simulink model "mech_cambelt"  (R2017b)
settings: Solver=ode5  StartTime=0.0  StopTime=5  FixedStep=0.01  RelTol=1e-3  EnableMultiTasking=on
undefined symbols (not defined in the file): m, rad, s, sigbuilder_block
libraries: mblibv1 x16
Description:
  | Cam Belt
  | 
  | This example shows a body rotating with a cam and a belt coupled to a pulley.
  | 
  | 
  | Copyright 2008-2017 The MathWorks, Inc.
settings Model: FPTRunName=Active  ExtModeAutoUpdateStatusClock=off  Creator=MathWorks  LastModifiedBy=smiller
settings DataIOCC: LimitDataPoints=on  SaveFormat=Array  SignalLoggingSaveFormat=ModelDataLogs  SignalLoggingName=sigsOut  OutputOption=SpecifiedOutputTimes  OutputTimes=[0:0.1:10]
settings OptimizationCC: ExpressionDepthLimit=2147483647  InitFltsAndDblsToZero=on  LifeSpan=inf
settings DebuggingCC: SaveWithParameterizedLinksMsg=none  UnderspecifiedInitializationDetection=Classic  MergeDetectMultiDrivingBlocksExec=none  CheckExecutionContextPreStartOutputMsg=on  CheckExecutionContextRuntimeOutputMsg=on  SignalResolutionControl=TryResolveAllWithWarning  MultiTaskDSMMsg=warning  MultiTaskCondExecSysMsg=none  SigSpecEnsureSampleTimeMsg=none  FcnCallInpInsideContextMsg=warning  StateNameClashWarn=warning  StrictBusMsg=None  SFUnexpectedBacktrackingDiag=warning  SFNoUnconditionalDefaultTransitionDiag=warning  SFExecutionAtInitializationDiag=none
settings HardwareCC: ProdBitPerPointer=32  ProdBitPerSizeT=32  ProdBitPerPtrDiffT=32  ProdLargestAtomicFloat=None  ProdIntDivRoundTo=Undefined  ProdEndianess=Unspecified  ProdWordSize=32  ProdHWDeviceType=32-bit Generic  TargetBitPerPointer=64  TargetBitPerSizeT=64  TargetBitPerPtrDiffT=64  TargetLongLongMode=on  TargetIntDivRoundTo=Zero  TargetEndianess=LittleEndian  TargetWordSize=64  TargetHWDeviceType=MATLAB Host  ProdEqTarget=off
settings ModelReferenceCC: PropagateSignalLabelsOutOfModel=off
settings RTWCC: Description=Generic Real-Time Target
settings CodeAppCC: StateflowObjectComments=on
settings GRTTargetCC: TargetLangStandard=C89/C90 (ANSI)  GeneratePreprocessorConditionals=Disable all  CombineOutputUpdateFcns=off  GRTInterface=on
settings ConfigComp: CovMetricSettings=dw  CovHtmlReporting=on  CovSaveCumulativeToWorkspaceVar=on  CovSaveSingleToWorkspaceVar=on  CovExternalEMLEnable=off
settings SimscapeCC: SimscapeNormalizeSystem=off
settings SimMechanicsCC: WarnOnRedundantConstraints=off  VisOnUpdateDiagram=on  VisDuringSimulation=on  VisConfigFile=mech_cambelt.mat
settings ConfigurationSet: Description=SimMechanics 2G

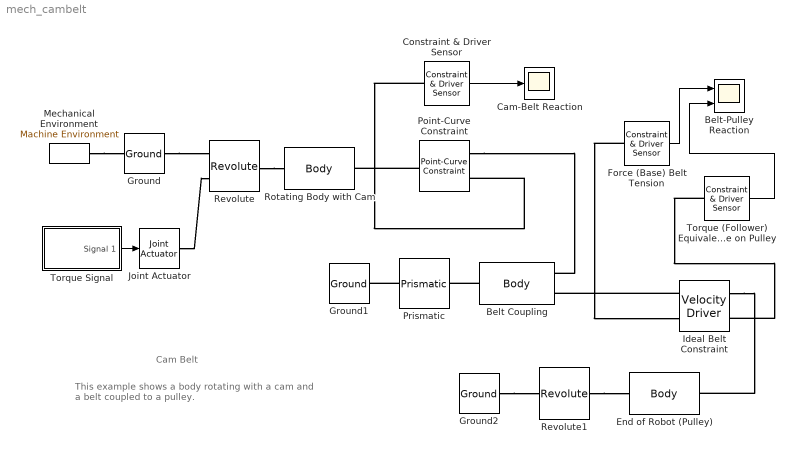
== system mech_cambelt ==
  note: Cam Belt
  note: This example shows a body rotating with a cam
      | and a belt coupled to a pulley.
  Belt Coupling : mblibv1/Bodies/Body  LConnTagsString=CS1  RConnTagsString=CS2|CS3  UpdateFromCAD=off  DialogClass=MechanicalBodyBlock  Mass=1  MassUnits=kg  InertiaUnits=kg*m^2  Inertia=(2/5)*1*[0.02 0 0;0 1 0;0 0 1]  Shape=Cylinder  ShapeDims=[1 1]  ShapeUnits=m  ShapeUse=false  Density=1  DensityUnits=kg/m^3  DensityUse=false  GraphicsMode=MACHINE_DEFAULT  BodyColorSelMode=MACHINE_DEFAULT  BodyColor=[1;0;0]  AttachedToCS=CG  CG=Left$CG$[2 0 0]$WORLD$WORLD$m$[0 0 0]$Euler X-Y-Z$deg$WORLD$false  WorkingFrames=Left$CS1$[3 0 0]$WORLD$WORLD$m$[0 0 0]$Euler X-Y-Z$deg$WORLD$true#Right$CS2$[1 0 0]$WORLD$WORLD$m$[0 0 0]$Euler X-Y-Z$deg$WORLD$true#Right$CS3$[1 0 0]$WORLD$WORLD$m$[0 0 0]$Euler X-Y-Z$deg$WORLD$true  CGPos=[2 0 0]  CGRot=[0 0 0]  CS0Pos=[]  CS0Rot=[]  CS1Pos=[3 0 0]  CS1Rot=[0 0 0]  CS2Pos=[1 0 0]  CS2Rot=[0 0 0]  CS3Pos=[1 0 0]  CS3Rot=[0 0 0]  CS4Pos=[]  CS4Rot=[]  CS5Pos=[]  CS5Rot=[]  CS6Pos=[]  CS6Rot=[]  CS7Pos=[]  CS7Rot=[]  CS8Pos=[]  CS8Rot=[]  CS9Pos=[]  CS9Rot=[]  CS10Pos=[]  CS10Rot=[]  CS11Pos=[]  CS11Rot=[]  CS12Pos=[]  CS12Rot=[]  CS13Pos=[]  CS13Rot=[]  CS14Pos=[]  CS14Rot=[]  CS15Pos=[]  CS15Rot=[]  CS16Pos=[]  CS16Rot=[]  CS17Pos=[]  CS17Rot=[]  CS18Pos=[]  CS18Rot=[]  CS19Pos=[]  CS19Rot=[]  CS20Pos=[]  CS20Rot=[]
      settings: SourceProductName=Simscape Multibody  SourceProductBaseCode=MS
  Belt-Pulley Reaction : Scope  NumInputPorts=2
  Cam-Belt Reaction : Scope
  Constraint & Driver Sensor : mblibv1/Sensors &  Actuators/Constraint & Driver  Sensor  UpdateFromCAD=off  LeftPortType=blob  RightPortType=blob  PhysicalDomain=Mechanical  DialogClass=ConstraintSensorBlock  SensedSide=Base  ReferenceFrame=Absolute (World)  ReactionForce=on  ForceUnits=N  ReactionMoment=on  MomentUnits=N-m  Muxed=on  OutputVector=[ 3 3 ]  ActiveIO=on  Width=6
      settings: SourceProductName=Simscape Multibody  SourceProductBaseCode=MS
  End of Robot (Pulley) : mblibv1/Bodies/Body  LConnTagsString=CS1  RConnTagsString=CS2  UpdateFromCAD=off  DialogClass=MechanicalBodyBlock  Mass=1  MassUnits=kg  InertiaUnits=kg*m^2  Inertia=(2/5)*1*[0.5 0 0;0 0.5 0;0 0 1]  Shape=Cylinder  ShapeDims=[1 1]  ShapeUnits=m  ShapeUse=false  Density=1  DensityUnits=kg/m^3  DensityUse=false  GraphicsMode=MACHINE_DEFAULT  BodyColorSelMode=MACHINE_DEFAULT  BodyColor=[1;0;0]  AttachedToCS=CG  CG=Left$CG$[0 0 0]$CS1$CS1$m$[0 0 0]$Euler X-Y-Z$deg$WORLD$false  WorkingFrames=Left$CS1$[0 0 0]$ADJOINING$ADJOINING$m$[0 0 0]$Euler X-Y-Z$deg$WORLD$true#Right$CS2$[0 0 0]$CS1$CS1$m$[0 0 0]$Euler X-Y-Z$deg$WORLD$true#Right$CS3$[0 1 0]$CS1$CS1$m$[0 0 0]$Euler X-Y-Z$deg$WORLD$false#Right$CS4$[-1 0 0]$CS1$CS1$m$[0 0 0]$Euler X-Y-Z$deg$WORLD$false#Right$CS5$[0 -1 0]$CS1$CS1$m$[0 0 0]$Euler X-Y-Z$deg$WORLD$false#Right$CS6$[1 0 0]$CS1$CS1$m$[0 0 0]$Euler X-Y-Z$deg$WORLD$false  CGPos=[0 0 0]  CGRot=[0 0 0]  CS0Pos=[]  CS0Rot=[]  CS1Pos=[0 0 0]  CS1Rot=[0 0 0]  CS2Pos=[0 0 0]  CS2Rot=[0 0 0]  CS3Pos=[0 1 0]  CS3Rot=[0 0 0]  CS4Pos=[-1 0 0]  CS4Rot=[0 0 0]  CS5Pos=[0 -1 0]  CS5Rot=[0 0 0]  CS6Pos=[1 0 0]  CS6Rot=[0 0 0]  CS7Pos=[]  CS7Rot=[]  CS8Pos=[]  CS8Rot=[]  CS9Pos=[]  CS9Rot=[]  CS10Pos=[]  CS10Rot=[]  CS11Pos=[]  CS11Rot=[]  CS12Pos=[]  CS12Rot=[]  CS13Pos=[]  CS13Rot=[]  CS14Pos=[]  CS14Rot=[]  CS15Pos=[]  CS15Rot=[]  CS16Pos=[]  CS16Rot=[]  CS17Pos=[]  CS17Rot=[]  CS18Pos=[]  CS18Rot=[]  CS19Pos=[]  CS19Rot=[]  CS20Pos=[]  CS20Rot=[]
      settings: SourceProductName=Simscape Multibody  SourceProductBaseCode=MS
  Force (Base) Belt Tension : mblibv1/Sensors &  Actuators/Constraint & Driver  Sensor  UpdateFromCAD=off  LeftPortType=blob  RightPortType=blob  PhysicalDomain=Mechanical  DialogClass=ConstraintSensorBlock  SensedSide=Base  ReferenceFrame=Absolute (World)  ReactionForce=on  ForceUnits=N  ReactionMoment=off  MomentUnits=N-m  Muxed=on  OutputVector=[ 3 ]  ActiveIO=on  Width=3
      settings: SourceProductName=Simscape Multibody  SourceProductBaseCode=MS
  Ground : mblibv1/Bodies/Ground  UpdateFromCAD=off  LeftPortType=env  RightPortType=workingframe  PhysicalDomain=Mechanical  DialogClass=GroundBlock  CoordPosition=[0 0 0]  CoordPositionUnits=m  StateVectorMgrId=-1  MachineId=[0 0]  ShowEnvPort=on  ParameterChecksum=[0 0 0 0]  TopologyChecksum=[0 0 0 0]
      settings: SourceProductName=Simscape Multibody  SourceProductBaseCode=MS
  Ground1 : mblibv1/Bodies/Ground  UpdateFromCAD=off  LeftPortType=env  RightPortType=workingframe  PhysicalDomain=Mechanical  DialogClass=GroundBlock  CoordPosition=[3 0 0]  CoordPositionUnits=m  StateVectorMgrId=-1  MachineId=[0 0]  ShowEnvPort=off  ParameterChecksum=[0 0 0 0]  TopologyChecksum=[0 0 0 0]
      settings: SourceProductName=Simscape Multibody  SourceProductBaseCode=MS
  Ground2 : mblibv1/Bodies/Ground  UpdateFromCAD=off  LeftPortType=env  RightPortType=workingframe  PhysicalDomain=Mechanical  DialogClass=GroundBlock  CoordPosition=[5 2 0]  CoordPositionUnits=m  StateVectorMgrId=-1  MachineId=[0 0]  ShowEnvPort=off  ParameterChecksum=[0 0 0 0]  TopologyChecksum=[0 0 0 0]
      settings: SourceProductName=Simscape Multibody  SourceProductBaseCode=MS
  Ideal Belt Constraint : mblibv1/Constraints &  Drivers/Velocity Driver  LConnTagsString=__newl0|SA1  RConnTagsString=__newr0|SA1  UpdateFromCAD=off  DialogClass=ConstantVelocityConstraint  NumSAPorts=2  Unit_V=m/s  Unit_Omega=rad/s  Coef_V_Base=[1 0 0]  Csys_V_Base=WORLD  Coef_Omega_Base=[0 0 0]  Csys_Omega_Base=WORLD  Coef_V_Follower=[0 0 0]  Csys_V_Follower=WORLD  Coef_Omega_Follower=[0 0 1]  Csys_Omega_Follower=WORLD
      settings: SourceProductName=Simscape Multibody  SourceProductBaseCode=MS
  Joint Actuator : mblibv1/Sensors &  Actuators/Joint Actuator  UpdateFromCAD=off  PhysicalDomain=Mechanical  PortType=blob  ActuationStyle=Force  AngleUnits=deg  ArcVelocityUnits=deg/s  ArcAccelerationUnits=deg/s^2  CoordPositionUnits=m  VelocityUnits=m/s  AccelerationUnits=m/s^2  ForceUnits=N  TorqueUnits=N-m  ActiveIO=on  Width=1  DialogClass=MechanicalActuatorBlock  Primitive=R1  ReferenceFrame=Absolute (INERTIAL)
      settings: SourceProductName=Simscape Multibody  SourceProductBaseCode=MS
  Mechanical Environment : mblibv1/Bodies/Machine Environment  Tag=Factory ground  PortType=env  PhysicalDomain=Mechanical  DialogTemplateClass=MECH.MachineEnvironment  SyncWhenCopied=off  Gravity=[0 -9.81 0]  GravityUnits=m/s^2  GravityAsSignal=off  Dimensionality=3D Only  AnalysisType=Forward dynamics  LinearAssemblyTolerance=1e-3  LinearAssemblyToleranceUnits=m  AngularAssemblyTolerance=1e-3  AngularAssemblyToleranceUnits=rad  ConstraintSolverType=Stabilizing  ConstraintRelTolerance=1e-4  ConstraintAbsTolerance=1e-4  UseRobustSingularityHandling=off  RedundancyAnalysisToleranceType=Automatically select tolerance  RedundancyAnalysisTolerance=1e-14  StatePerturbationType=Fixed  PerturbationSize=1e-5  VisualizeMachine=on  BodyVisualizationType=Use model default body geometries  BodyColorSelMode=Use model default  DefaultBodyColor=[1 0 0]
      settings: SourceProductName=Simscape Multibody  SourceProductBaseCode=MS
  Point-Curve Constraint : mblibv1/Constraints &  Drivers/Point-Curve Constraint  LConnTagsString=__newl0|SA1  RConnTagsString=__newr0  UpdateFromCAD=off  DialogClass=PointCurveConstraint  Units=m  Xbreaks="[1     0.77547    0.058989    -0.52528    -0.55899    -0.17022     0.65485]"  Ybreaks="[0     0.42955     0.56832     0.29503    -0.12733    -0.36512    -0.39199]"  Zbreaks="[-0.0031056     0.36957     0.56832     0.29503    -0.12733    -0.46273    -0.40062]*0"  EndConditions=periodic  CanExtrapolate=off  NumSAPorts=1
      settings: SourceProductName=Simscape Multibody  SourceProductBaseCode=MS
  Prismatic : mblibv1/Joints/Prismatic  LConnTagsString=__newl0  RConnTagsString=__newr0  UpdateFromCAD=off  NumSAPorts=0  CutJoint=off  MarkAsCut=off  Primitives=prismatic  PrimitiveProps=P1$WORLD$[-1 0 0]$prismatic  DialogClass=JointBlock  P1Axis=[-1 0 0]
      settings: SourceProductName=Simscape Multibody  SourceProductBaseCode=MS
  Revolute : mblibv1/Joints/Revolute  LConnTagsString=__newl0|SA1  RConnTagsString=__newr0  UpdateFromCAD=off  NumSAPorts=1  CutJoint=off  MarkAsCut=off  Primitives=revolute  PrimitiveProps=R1$WORLD$[0 0 1]$revolute  DialogClass=JointBlock  R1Axis=[0 0 1]
      settings: SourceProductName=Simscape Multibody  SourceProductBaseCode=MS
  Revolute1 : mblibv1/Joints/Revolute  LConnTagsString=__newl0  RConnTagsString=__newr0  UpdateFromCAD=off  NumSAPorts=0  CutJoint=off  MarkAsCut=off  Primitives=revolute  PrimitiveProps=R1$WORLD$[0 0 1]$revolute  DialogClass=JointBlock  R1Axis=[0 0 1]
      settings: SourceProductName=Simscape Multibody  SourceProductBaseCode=MS
  Rotating Body with Cam : mblibv1/Bodies/Body  LConnTagsString=CS1  RConnTagsString=CS2  UpdateFromCAD=off  DialogClass=MechanicalBodyBlock  Mass=1  MassUnits=kg  InertiaUnits=kg*m^2  Inertia=(2/5)*1*[0.5 0 0;0 0.5 0;0 0 1]  Shape=Cylinder  ShapeDims=[1 1]  ShapeUnits=m  ShapeUse=false  Density=1  DensityUnits=kg/m^3  DensityUse=false  GraphicsMode=MACHINE_DEFAULT  BodyColorSelMode=MACHINE_DEFAULT  BodyColor=[1;0;0]  AttachedToCS=CG  CG=Left$CG$[0 0 0]$WORLD$WORLD$m$[0 0 0]$Euler X-Y-Z$deg$WORLD$false  WorkingFrames=Left$CS1$[0 0 0]$WORLD$WORLD$m$[0 0 0]$Euler X-Y-Z$deg$WORLD$true#Right$CS2$[0 0 0]$CS1$CS1$m$[0 0 0]$Euler X-Y-Z$deg$WORLD$true#Right$CS3$[0 1 0]$CS1$CS1$m$[0 0 0]$Euler X-Y-Z$deg$WORLD$false#Right$CS4$[-1 0 0]$CS1$CS1$m$[0 0 0]$Euler X-Y-Z$deg$WORLD$false#Right$CS5$[0 -1 0]$CS1$CS1$m$[0 0 0]$Euler X-Y-Z$deg$WORLD$false#Right$CS6$[1 0 0]$CS1$CS1$m$[0 0 0]$Euler X-Y-Z$deg$WORLD$false  CGPos=[0 0 0]  CGRot=[0 0 0]  CS0Pos=[]  CS0Rot=[]  CS1Pos=[0 0 0]  CS1Rot=[0 0 0]  CS2Pos=[0 0 0]  CS2Rot=[0 0 0]  CS3Pos=[0 1 0]  CS3Rot=[0 0 0]  CS4Pos=[-1 0 0]  CS4Rot=[0 0 0]  CS5Pos=[0 -1 0]  CS5Rot=[0 0 0]  CS6Pos=[1 0 0]  CS6Rot=[0 0 0]  CS7Pos=[]  CS7Rot=[]  CS8Pos=[]  CS8Rot=[]  CS9Pos=[]  CS9Rot=[]  CS10Pos=[]  CS10Rot=[]  CS11Pos=[]  CS11Rot=[]  CS12Pos=[]  CS12Rot=[]  CS13Pos=[]  CS13Rot=[]  CS14Pos=[]  CS14Rot=[]  CS15Pos=[]  CS15Rot=[]  CS16Pos=[]  CS16Rot=[]  CS17Pos=[]  CS17Rot=[]  CS18Pos=[]  CS18Rot=[]  CS19Pos=[]  CS19Rot=[]  CS20Pos=[]  CS20Rot=[]
      settings: SourceProductName=Simscape Multibody  SourceProductBaseCode=MS
  Torque Signal : Subsystem  Tag=STV Subsys  LoadFcn=sigbuilder_block('load');  StartFcn=sigbuilder_block('start');  StopFcn=sigbuilder_block('stop');  ClipboardFcn=sigbuilder_block('clipboard');  mask(Sigbuilder block){tuvar=[0:10]}
      mask help: Sigbuilder GUI
      mask init:
      | if ~strcmp(get_param(bdroot,'SimulationStatus'),'stopped') tuvar = sigbuilder_block('maskInit'); end
      settings: CopyFcn=sigbuilder_block('copy');  DeleteFcn=sigbuilder_block('delete');  ModelCloseFcn=sigbuilder_block('modelClose');  PreSaveFcn=sigbuilder_block('preSave');  PauseFcn=sigbuilder_block('pause')  ContinueFcn=sigbuilder_block('continue')  NameChangeFcn=sigbuilder_block('namechange');  OpenFcn=sigbuilder_block('open',[57 48.75 519.75 399.75 ]);  CloseFcn=sigbuilder_block('close');
      mask Display: plot(0, 0, 100, 100,[2, 2, 32, 32, 2], [68, 8, 8, 68, 68],[32, 2], [38, 38], [32, 19, 2],[53, 60, 44], [32, 17, 17, 2],[16, 16, 31, 31]);txt = getActiveGroup(gcbh);text(2, 100, txt,'verticalAlignment', 'top');
  Torque (Follower) Equivalent Torque on Pulley : mblibv1/Sensors &  Actuators/Constraint & Driver  Sensor  UpdateFromCAD=off  LeftPortType=blob  RightPortType=blob  PhysicalDomain=Mechanical  DialogClass=ConstraintSensorBlock  SensedSide=Follower  ReferenceFrame=Absolute (World)  ReactionForce=off  ForceUnits=N  ReactionMoment=on  MomentUnits=N-m  Muxed=on  OutputVector=[ 3 ]  ActiveIO=on  Width=3
      settings: SourceProductName=Simscape Multibody  SourceProductBaseCode=MS
  wires:
  Torque Signal/1(Signal 1) -> Joint Actuator/1
  Constraint & Driver Sensor/1 -> Cam-Belt Reaction/1
  Torque (Follower) Equivalent Torque on Pulley/1 -> Belt-Pulley Reaction/2
  Force (Base) Belt Tension/1 -> Belt-Pulley Reaction/1
  connections:
  Ground/RConn1 -- Revolute/LConn1
  Revolute/RConn1 -- Rotating Body with Cam/LConn1
  Joint Actuator/RConn1 -- Revolute/LConn2
  Prismatic/LConn1 -- Ground1/RConn1
  Belt Coupling/LConn1 -- Prismatic/RConn1
  Point-Curve Constraint/LConn1 -- Belt Coupling/RConn1
  Point-Curve Constraint/RConn1 -- Rotating Body with Cam/RConn1
  Constraint & Driver Sensor/LConn1 -- Point-Curve Constraint/LConn2
  Ground2/RConn1 -- Revolute1/LConn1
  Revolute1/RConn1 -- End of Robot (Pulley)/LConn1
  Ideal Belt Constraint/RConn1 -- End of Robot (Pulley)/RConn1
  Ideal Belt Constraint/LConn1 -- Belt Coupling/RConn2
  Force (Base) Belt Tension/LConn1 -- Ideal Belt Constraint/LConn2
  Torque (Follower) Equivalent Torque on Pulley/LConn1 -- Ideal Belt Constraint/RConn2
  Mechanical Environment/RConn1 -- Ground/LConn1

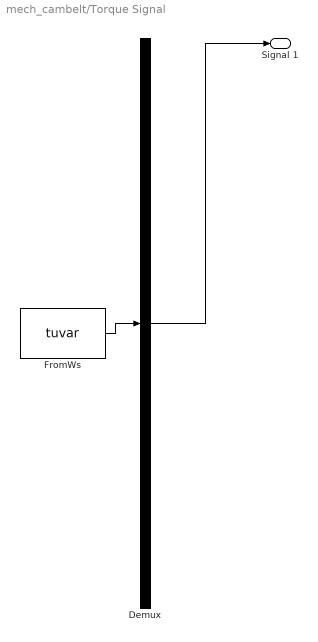
== system mech_cambelt/Torque Signal ==
  Demux : Demux  Tag=STV Demux  Outputs=1
  FromWs : FromWorkspace  Tag=STV FromWs  VariableName=tuvar  SampleTime=0
      SigBuilderData=|
      | dataSet.timeRange = [0 10]
      | dataSet.name = 'Group 1'
      | sbobj.Groups.Name = 'Group 1'
      | sbobj.Groups.Signals.Name = 'Signal 1'
      | sbobj.Groups.Signals.XData = [0 0.58 0.58 1.16 1.94 1.94 10]
      | sbobj.Groups.Signals.YData = [0 0 0.12 4.81 0.2 0.02 -0.12]
  Signal 1 : Outport  Tag=STV Outport
  wires:
  Demux/1 -> Signal 1/1
  FromWs/1 -> Demux/1
